simulink model "q2"  (R2023a)
settings: Solver=VariableStepAuto  StartTime=0.0  StopTime=1  RelTol=1e-3
libraries: dspsnks4 x1, dspvision x1, dspsigops x1
settings Model: Creator=J_MEHMAN  LastModifiedBy=J_MEHMAN

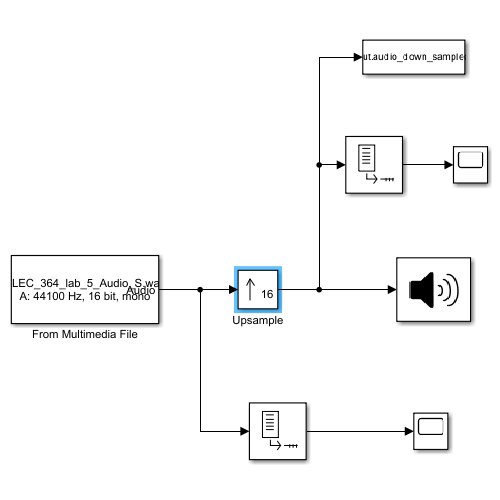
[thumbnail: Simulink's stored preview of the top-level diagram]
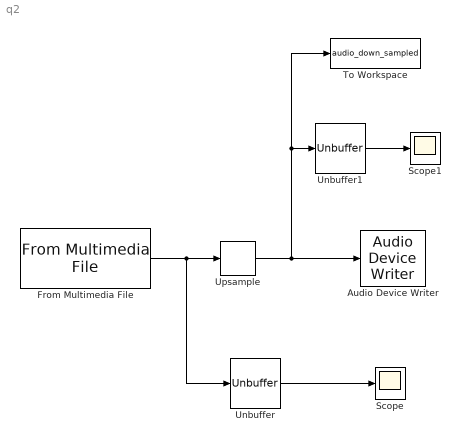
== system q2 ==
  Audio Device Writer : dspsnks4/Audio Device Writer  Driver=DirectSound  Device=Speakers (Realtek(R) Audio)  InheritSampleRate=off  SampleRate=44100  BitDepth=16-bit integer  BufferSize=4096  NumBuffers=10  DefaultOutputChannelMapping=on  OutputChannelMapping=1:2  OutputNumUnderrunSamples=off  DriverIdx=1  DeviceWarnFlag=''
  From Multimedia File : dspvision/From Multimedia File  inputFilename=U:\elec_342\lab 4\ELEC_364_lab_5_Audio_S.wav  readRange=[1 Inf]  loop=on  numPlays=inf  outputStreams=Audio only  videoDataType=single  audioDataType=double  inheritSampleTime=on  userDefinedSampleTime=1/30  noAudioOutput=off  isIntensityVideo=off  fourcc=RGB  colorVideoFormat=Separate color signals  outputEOF=off  dataOrg=Column-major  audioFrameSize=1024  computeAudioFrameSize=off  outSamplingMode=Sample based
      settings: LibrarySourceBlock=dspsrcs4/From Multimedia File
  Scope : Scope
  Scope1 : Scope
  To Workspace : ToWorkspace  VariableName=audio_down_sampled  SampleTime=-1
      settings: Save2DSignal=2-D array (concatenate along first dimension)
  Unbuffer : Unbuffer
  Unbuffer1 : Unbuffer
  Upsample : dspsigops/Upsample  FactorSource=Dialog parameter  N=16  Nmax=16  phase=0  RateOptions=Allow multirate processing  ic=0  mode=Unused parameter value
      settings: LibrarySourceBlock=dsphdlsupportsigops/Upsample
  wires:
  From Multimedia File/1 -> Upsample/1, Unbuffer/1
  Upsample/1 -> To Workspace/1, Unbuffer1/1, Audio Device Writer/1
  Unbuffer/1 -> Scope/1
  Unbuffer1/1 -> Scope1/1
